simulink model "wending_machine"  (R2019b)
settings: Solver=FixedStepDiscrete  StartTime=0.0  StopTime=10.0  FixedStep=1  RelTol=1e-3
settings Model: Creator=dell  LastModifiedBy=dell
settings SFSimCC: CustomCodeUndefinedFunction=UseInterfaceOnly

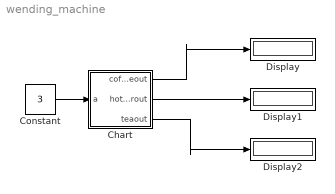
== system wending_machine ==
  Chart : Stateflow chart  BlockKeywords=__PRM__SERIALIZED__DATA__:Stateflow Chart,Stateflow Diagram  TreatAsAtomicUnit=on
  Constant : Constant  Value=3
  Display : Display
  Display1 : Display
  Display2 : Display
  wires:
  Chart/1(coffeeout) -> Display/1
  Chart/2(hotwaterout) -> Display1/1
  Constant/1 -> Chart/1(a)
  Chart/3(teaout) -> Display2/1

== stateflow chart wending_machine/Chart ==
  state coffee
    coffeeout=1;
    teaout=0;
    hotwaterout=0;
  note: wending machine
  note: when ip 1 : coffee on(1) for 5 sec
      | when ip 2 : tea on(1) for 5 sec
      | when ip 3 : hot water on(1) for 5 sec
  state input
    coffeeout=0;
    teaout=0;
    hotwater=0;
  state tea
    teaout=1;
    coffeeout=0;
    hotwaterout=0;
  state hotwater
    hotwaterout=1;
    teaout=0;
    coffee=0;
  coffee -> input : after(5,sec)
  (junction 6) -> coffee [order 1] : [a==1]
  (default) -> input
  input -> (junction 6)
  (junction 6) -> tea [order 2] : [a==2]
  (junction 6) -> hotwater [order 3] : [a==3]
  tea -> input : after(5,sec)
  hotwater -> input : after(5,sec)
  data: a input; coffeeout output; hotwaterout output; teaout output; coffee local; hotwater local
